simulink model "model_quarter_car_BG"  (Simulink 7.5)
settings: Solver=ode4  StartTime=0.0  StopTime=10  FixedStep=0.005  MaxStep=1e-6  RelTol=1e-3
settings Model: Creator=Slim  LastModifiedBy=Slim

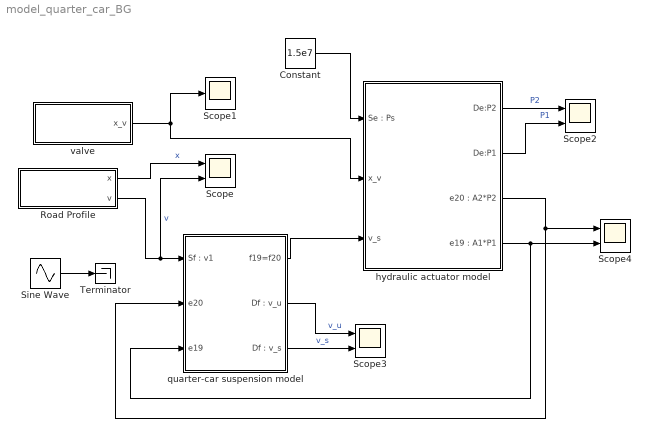
== system model_quarter_car_BG ==
  Constant : Constant  Value=1.5e7  OutDataType=fixdt(1, 16)  OutScaling=2^0
  Road Profile : Subsystem
  Scope{,2..4} (4 alike) : Scope  NumInputPorts=2
      Scope settings: YMin=-1~-5  YMax=1~5
      Scope2 settings: YMin=-1.25e+007~-5  YMax=1.25e+007~5  SaveName=ScopeData2
      Scope3 settings: YMin=-5~-5  YMax=5~5  SaveName=ScopeData3
      Scope4 settings: YMin=-1.25e+007~-5  YMax=1.25e+007~5  SaveName=ScopeData5
  Scope1 : Scope
      settings: YMin=6.25e-037  YMax=8.75e-037
  Sine Wave : Sin  Amplitude=0.08*pi  Bias=0  Frequency=2*pi  Phase=pi/2  Samples=10  SampleTime=0  Offset=0
  Terminator : Terminator
  hydraulic actuator model : Subsystem
  quarter-car suspension model : Subsystem
  valve : Subsystem
  wires:
  hydraulic actuator model/4("e19 : A1*P1") -> quarter-car suspension model/3(e19), Scope4/2
  hydraulic actuator model/3("e20 : A2*P2") -> quarter-car suspension model/2(e20), Scope4/1
  Road Profile/1(x) -> Scope/1  "x"
  valve/1(x_v) -> Scope1/1, hydraulic actuator model/2(x_v)
  Constant/1 -> hydraulic actuator model/1("Se : Ps")
  quarter-car suspension model/1(f19=f20) -> hydraulic actuator model/3(v_s)
  quarter-car suspension model/2("Df : v_u") -> Scope3/1  "v_u"
  quarter-car suspension model/3("Df : v_s") -> Scope3/2  "v_s"
  hydraulic actuator model/1(De:P2) -> Scope2/1  "P2"
  hydraulic actuator model/2(De:P1) -> Scope2/2  "P1"
  Sine Wave/1 -> Terminator/1
  Road Profile/2(v) -> quarter-car suspension model/1("Sf : v1"), Scope/2  "v"

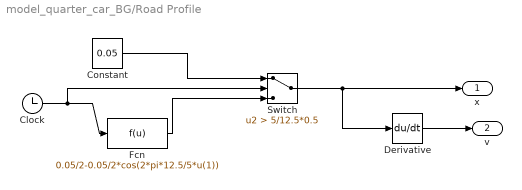
== system model_quarter_car_BG/Road Profile ==
  Clock : Clock
      settings: Decimation=10
  Constant : Constant  Value=0.05  OutDataType=fixdt(1, 16)  OutScaling=2^0
  Derivative : Derivative
  Fcn : Fcn  Expr=0.05/2-0.05/2*cos(2*pi*12.5/5*u(1))
  Switch : Switch  Criteria=u2 > Threshold  Threshold=5/12.5*0.5  OutDataType=fixdt(1, 16)  OutScaling=2^0
  x : Outport  OutDataType=fixdt(1, 16)  OutScaling=2^0
  v : Outport  Port=2  OutDataType=fixdt(1, 16)  OutScaling=2^0
  wires:
  Clock/1 -> Fcn/1, Switch/2
  Constant/1 -> Switch/1
  Fcn/1 -> Switch/3
  Switch/1 -> x/1, Derivative/1
  Derivative/1 -> v/1

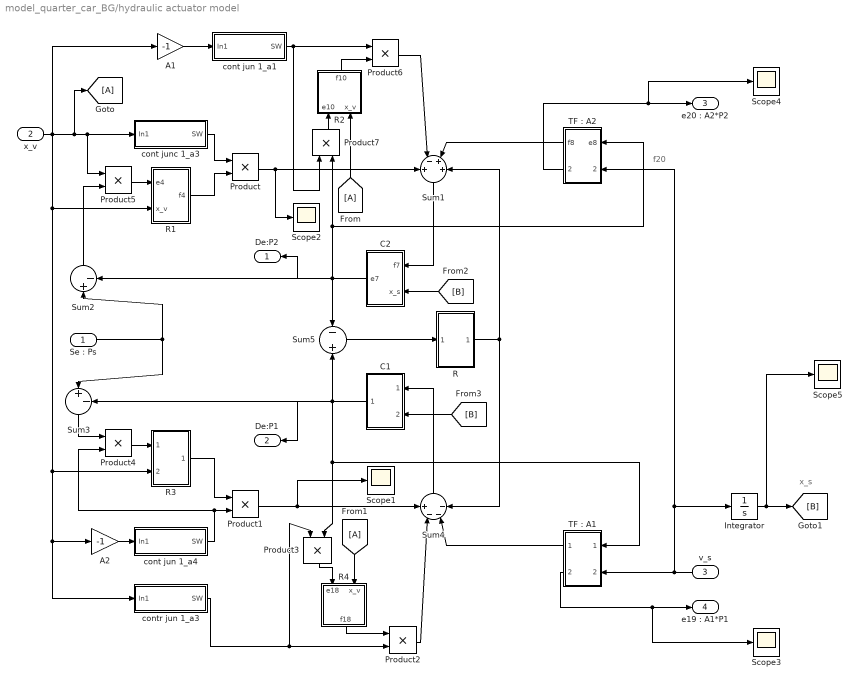
== system model_quarter_car_BG/hydraulic actuator model ==
  note: f20
  note: x_s
  "Se : Ps" : Inport  OutDataType=fixdt(1, 16)  OutScaling=2^0
  x_v : Inport  Port=2  OutDataType=fixdt(1, 16)  OutScaling=2^0
  v_s : Inport  Port=3  OutDataType=fixdt(1, 16)  OutScaling=2^0
  A1 : Gain  Gain=-1  ParameterDataType=fixdt(1, 16)  ParameterScaling=2^0  OutDataType=fixdt(1, 16)  OutScaling=2^0
  A2 : Gain  Gain=-1  ParameterDataType=fixdt(1, 16)  ParameterScaling=2^0  OutDataType=fixdt(1, 16)  OutScaling=2^0
  C1 : Subsystem
  C2 : Subsystem
  Integrator : Integrator
  Product{,1..7} (8 alike) : Product  OutDataType=fixdt(1, 16)  OutScaling=2^0  RndMeth=Zero
  R : Subsystem
  R1 : Subsystem
  R2 : Subsystem
  R3 : Subsystem
  R4 : Subsystem
  Scope{1..5} (5 alike) : Scope
      Scope1 settings: YMin=-1.25e+007  YMax=1.25e+007  SaveName=ScopeData6
      Scope2 settings: YMin=-1.25e+007  YMax=1.25e+007  SaveName=ScopeData4
      Scope3 settings: YMin=-1.25e+007  YMax=1.25e+007  SaveName=ScopeData8
      Scope4 settings: YMin=-1.25e+007  YMax=1.25e+007  SaveName=ScopeData9
      Scope5 settings: YMin=-1.25e+007  YMax=1.25e+007  SaveName=ScopeData10
  Sum1 : Sum  Inputs=+-++  OutDataType=fixdt(1, 16)  OutScaling=2^0
  Sum2 : Sum  Inputs=|+-  OutDataType=fixdt(1, 16)  OutScaling=2^0
  Sum3 : Sum  Inputs=|+-  OutDataType=fixdt(1, 16)  OutScaling=2^0
  Sum4 : Sum  Inputs=+---  OutDataType=fixdt(1, 16)  OutScaling=2^0
  Sum5 : Sum  Inputs=-+  OutDataType=fixdt(1, 16)  OutScaling=2^0
  "TF : A1" : Subsystem
  "TF : A2" : Subsystem
  cont jun 1_a1 : Subsystem
  cont jun 1_a4 : Subsystem
  cont junc 1_a3 : Subsystem
  contr jun 1_a3 : Subsystem
  De:P2 : Outport  OutDataType=fixdt(1, 16)  OutScaling=2^0
  De:P1 : Outport  Port=2  OutDataType=fixdt(1, 16)  OutScaling=2^0
  "e20 : A2*P2" : Outport  Port=3  OutDataType=fixdt(1, 16)  OutScaling=2^0
  "e19 : A1*P1" : Outport  Port=4  OutDataType=fixdt(1, 16)  OutScaling=2^0
  wires:
  "Se : Ps"/1 -> Sum2/1, Sum3/1
  cont junc 1_a3/1(SW) -> Product/1
  R1/1(f4) -> Product/2
  C2/1(e7) -> Sum2/2, Sum5/1, De:P2/1, "TF : A2"/1(e8), Product7/2
  Sum1/1 -> C2/1(f7)
  cont jun 1_a4/1(SW) -> Product1/2, Product4/2
  R3/1(f14) -> Product1/1
  Product/1 -> Sum1/1, Scope2/1
  C1/1(e16) -> Sum3/2, Sum5/2, De:P1/1, "TF : A1"/1(e17), Product3/2
  Sum4/1 -> C1/1(f16)
  Sum5/1 -> R/1(e11)
  Product1/1 -> Sum4/1, Scope1/1
  R/1(f11) -> Sum1/4, Sum4/4
  "TF : A2"/1(f8) -> Sum1/3
  "TF : A1"/1(f17) -> Sum4/3
  v_s/1 -> "TF : A1"/2(f19), "TF : A2"/2(f20), Integrator/1
  "TF : A1"/2(e19) -> "e19 : A1*P1"/1, Scope3/1
  "TF : A2"/2(e20) -> "e20 : A2*P2"/1, Scope4/1
  x_v/1 -> [A], cont junc 1_a3/1(In1), Product5/1, R3/2(x_v), A2/1, contr jun 1_a3/1(In1), R1/2(x_v), A1/1
  A2/1 -> cont jun 1_a4/1(In1)
  [A] -> R2/2(x_v)
  [A] -> R4/2(x_v)
  Integrator/1 -> [B], Scope5/1
  [B] -> C2/2(x_s)
  [B] -> C1/2(x_s)
  Sum2/1 -> Product5/2
  Sum3/1 -> Product4/1
  contr jun 1_a3/1(SW) -> Product2/2, Product3/1
  R4/1(f18) -> Product2/1
  Product2/1 -> Sum4/2
  Product3/1 -> R4/1(e18)
  Product4/1 -> R3/1(e14)
  Product5/1 -> R1/1(e4)
  A1/1 -> cont jun 1_a1/1(In1)
  cont jun 1_a1/1(SW) -> Product6/1, Product7/1
  R2/1(f10) -> Product6/2
  Product6/1 -> Sum1/2
  Product7/1 -> R2/1(e10)

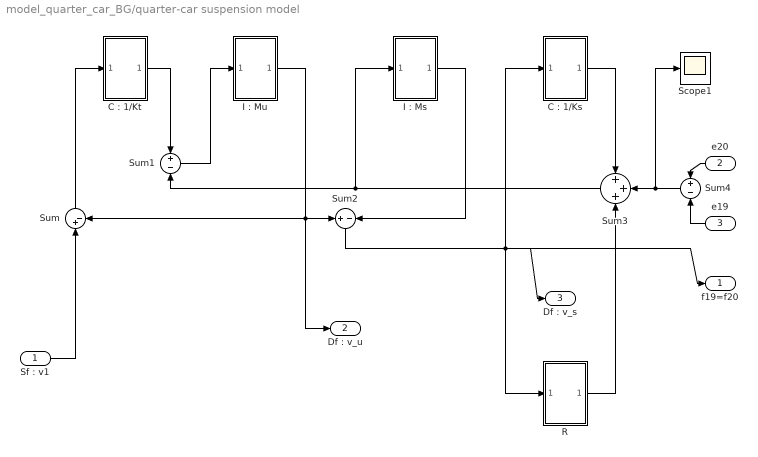
== system model_quarter_car_BG/quarter-car suspension model ==
  "Sf : v1" : Inport  OutDataType=fixdt(1, 16)  OutScaling=2^0
  e20 : Inport  Port=2  OutDataType=fixdt(1, 16)  OutScaling=2^0
  e19 : Inport  Port=3  OutDataType=fixdt(1, 16)  OutScaling=2^0
  "C : 1/Ks" : Subsystem
  "C : 1/Kt" : Subsystem
  "I : Ms" : Subsystem
  "I : Mu" : Subsystem
  R : Subsystem
  Scope1 : Scope
      settings: YMin=6.25e-037  YMax=8.75e-037  SaveName=ScopeData11
  Sum : Sum  Inputs=|+-  OutDataType=fixdt(1, 16)  OutScaling=2^0
  Sum1 : Sum  Inputs=+-  OutDataType=fixdt(1, 16)  OutScaling=2^0
  Sum2 : Sum  Inputs=+-  OutDataType=fixdt(1, 16)  OutScaling=2^0
  Sum3 : Sum  Inputs=+++  OutDataType=fixdt(1, 16)  OutScaling=2^0
  Sum4 : Sum  Inputs=+-  OutDataType=fixdt(1, 16)  OutScaling=2^0
  f19=f20 : Outport  OutDataType=fixdt(1, 16)  OutScaling=2^0
  "Df : v_u" : Outport  Port=2  OutDataType=fixdt(1, 16)  OutScaling=2^0
  "Df : v_s" : Outport  Port=3  OutDataType=fixdt(1, 16)  OutScaling=2^0
  wires:
  "Sf : v1"/1 -> Sum/1
  Sum/1 -> "C : 1/Kt"/1(f28)
  "C : 1/Kt"/1(e28) -> Sum1/1
  Sum1/1 -> "I : Mu"/1(e26)
  "I : Mu"/1(f26) -> Sum2/1, Sum/2, "Df : v_u"/1
  "I : Ms"/1(f24) -> Sum2/2
  Sum3/1 -> Sum1/2, "I : Ms"/1(e24)
  Sum2/1 -> "C : 1/Ks"/1(f21), R/1(f23), f19=f20/1, "Df : v_s"/1
  "C : 1/Ks"/1(e21) -> Sum3/1
  R/1(e23) -> Sum3/3
  e19/1 -> Sum4/2
  e20/1 -> Sum4/1
  Sum4/1 -> Sum3/2, Scope1/1

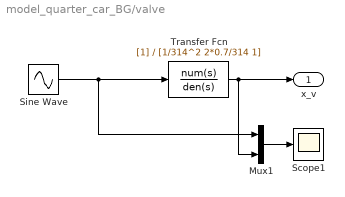
== system model_quarter_car_BG/valve ==
  Mux1 : Mux  Inputs=2
  Scope1 : Scope
      settings: YMin=6.25e-037  YMax=8.75e-037  SaveName=ScopeData7
  Sine Wave : Sin  Amplitude=2  Bias=0  Frequency=pi  Phase=0  Samples=10  SampleTime=0  Offset=0
  Transfer Fcn : TransferFcn  Denominator=[1/314^2 2*0.7/314 1]
  x_v : Outport  OutDataType=fixdt(1, 16)  OutScaling=2^0
  wires:
  Transfer Fcn/1 -> x_v/1, Mux1/2
  Sine Wave/1 -> Transfer Fcn/1, Mux1/1
  Mux1/1 -> Scope1/1

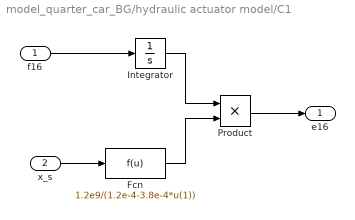
== system model_quarter_car_BG/hydraulic actuator model/C1 ==
  f16 : Inport  OutDataType=fixdt(1, 16)  OutScaling=2^0
  x_s : Inport  Port=2  OutDataType=fixdt(1, 16)  OutScaling=2^0
  Fcn : Fcn  Expr=1.2e9/(1.2e-4-3.8e-4*u(1))
  Integrator : Integrator
  Product : Product  OutDataType=fixdt(1, 16)  OutScaling=2^0  RndMeth=Zero
  e16 : Outport  OutDataType=fixdt(1, 16)  OutScaling=2^0
  wires:
  f16/1 -> Integrator/1
  Integrator/1 -> Product/1
  x_s/1 -> Fcn/1
  Fcn/1 -> Product/2
  Product/1 -> e16/1

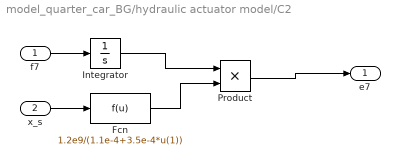
== system model_quarter_car_BG/hydraulic actuator model/C2 ==
  f7 : Inport  OutDataType=fixdt(1, 16)  OutScaling=2^0
  x_s : Inport  Port=2  OutDataType=fixdt(1, 16)  OutScaling=2^0
  Fcn : Fcn  Expr=1.2e9/(1.1e-4+3.5e-4*u(1))
  Integrator : Integrator
  Product : Product  OutDataType=fixdt(1, 16)  OutScaling=2^0  RndMeth=Zero
  e7 : Outport  OutDataType=fixdt(1, 16)  OutScaling=2^0
  wires:
  x_s/1 -> Fcn/1
  f7/1 -> Integrator/1
  Integrator/1 -> Product/1
  Fcn/1 -> Product/2
  Product/1 -> e7/1

== system model_quarter_car_BG/hydraulic actuator model/R ==
  e11 : Inport  OutDataType=fixdt(1, 16)  OutScaling=2^0
  1/Ctm : Gain  Gain=0.3e-12  ParameterDataType=fixdt(1, 16)  ParameterScaling=2^0  OutDataType=fixdt(1, 16)  OutScaling=2^0
  f11 : Outport  OutDataType=fixdt(1, 16)  OutScaling=2^0
  wires:
  e11/1 -> 1/Ctm/1
  1/Ctm/1 -> f11/1

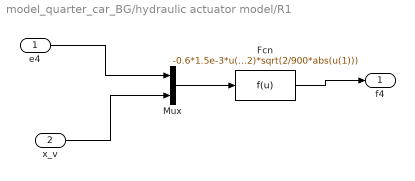
== system model_quarter_car_BG/hydraulic actuator model/R1 ==
  e4 : Inport  OutDataType=fixdt(1, 16)  OutScaling=2^0
  x_v : Inport  Port=2  OutDataType=fixdt(1, 16)  OutScaling=2^0
  Fcn : Fcn  Expr=-0.6*1.5e-3*u(2)*sqrt(2/900*abs(u(1)))
  Mux : Mux  Inputs=2
  f4 : Outport  OutDataType=fixdt(1, 16)  OutScaling=2^0
  wires:
  x_v/1 -> Mux/2
  e4/1 -> Mux/1
  Mux/1 -> Fcn/1
  Fcn/1 -> f4/1

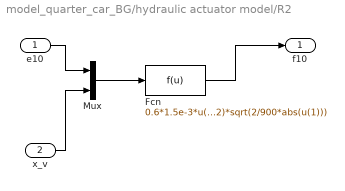
== system model_quarter_car_BG/hydraulic actuator model/R2 ==
  e10 : Inport  OutDataType=fixdt(1, 16)  OutScaling=2^0
  x_v : Inport  Port=2  OutDataType=fixdt(1, 16)  OutScaling=2^0
  Fcn : Fcn  Expr=0.6*1.5e-3*u(2)*sqrt(2/900*abs(u(1)))
  Mux : Mux  Inputs=2
  f10 : Outport  OutDataType=fixdt(1, 16)  OutScaling=2^0
  wires:
  e10/1 -> Mux/1
  x_v/1 -> Mux/2
  Mux/1 -> Fcn/1
  Fcn/1 -> f10/1

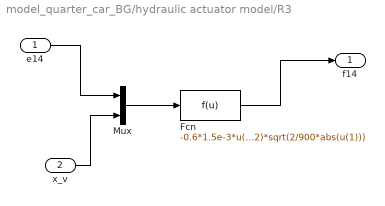
== system model_quarter_car_BG/hydraulic actuator model/R3 ==
  e14 : Inport  OutDataType=fixdt(1, 16)  OutScaling=2^0
  x_v : Inport  Port=2  OutDataType=fixdt(1, 16)  OutScaling=2^0
  Fcn : Fcn  Expr=-0.6*1.5e-3*u(2)*sqrt(2/900*abs(u(1)))
  Mux : Mux  Inputs=2
  f14 : Outport  OutDataType=fixdt(1, 16)  OutScaling=2^0
  wires:
  Mux/1 -> Fcn/1
  Fcn/1 -> f14/1
  e14/1 -> Mux/1
  x_v/1 -> Mux/2

== system model_quarter_car_BG/hydraulic actuator model/R4 ==
  e18 : Inport  OutDataType=fixdt(1, 16)  OutScaling=2^0
  x_v : Inport  Port=2  OutDataType=fixdt(1, 16)  OutScaling=2^0
  Fcn : Fcn  Expr=0.6*1.5e-3*u(2)*sqrt(2/900*abs(u(1)))
  Mux : Mux  Inputs=2
  f18 : Outport  OutDataType=fixdt(1, 16)  OutScaling=2^0
  wires:
  Fcn/1 -> f18/1
  Mux/1 -> Fcn/1
  e18/1 -> Mux/1
  x_v/1 -> Mux/2

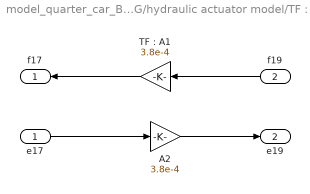
== system model_quarter_car_BG/hydraulic actuator model/TF : A1 ==
  e17 : Inport  OutDataType=fixdt(1, 16)  OutScaling=2^0
  f19 : Inport  Port=2  OutDataType=fixdt(1, 16)  OutScaling=2^0
  A2 : Gain  Gain=3.8e-4  ParameterDataType=fixdt(1, 16)  ParameterScaling=2^0  OutDataType=fixdt(1, 16)  OutScaling=2^0
  "TF : A1" : Gain  Gain=3.8e-4  ParameterDataType=fixdt(1, 16)  ParameterScaling=2^0  OutDataType=fixdt(1, 16)  OutScaling=2^0
  f17 : Outport  OutDataType=fixdt(1, 16)  OutScaling=2^0
  e19 : Outport  Port=2  OutDataType=fixdt(1, 16)  OutScaling=2^0
  wires:
  A2/1 -> e19/1
  e17/1 -> A2/1
  "TF : A1"/1 -> f17/1
  f19/1 -> "TF : A1"/1

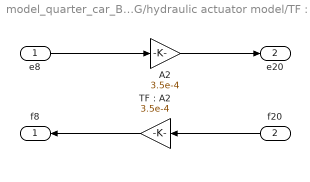
== system model_quarter_car_BG/hydraulic actuator model/TF : A2 ==
  e8 : Inport  OutDataType=fixdt(1, 16)  OutScaling=2^0
  f20 : Inport  Port=2  OutDataType=fixdt(1, 16)  OutScaling=2^0
  A2 : Gain  Gain=3.5e-4  ParameterDataType=fixdt(1, 16)  ParameterScaling=2^0  OutDataType=fixdt(1, 16)  OutScaling=2^0
  "TF : A2" : Gain  Gain=3.5e-4  ParameterDataType=fixdt(1, 16)  ParameterScaling=2^0  OutDataType=fixdt(1, 16)  OutScaling=2^0
  f8 : Outport  OutDataType=fixdt(1, 16)  OutScaling=2^0
  e20 : Outport  Port=2  OutDataType=fixdt(1, 16)  OutScaling=2^0
  wires:
  f20/1 -> "TF : A2"/1
  "TF : A2"/1 -> f8/1
  e8/1 -> A2/1
  A2/1 -> e20/1

== system model_quarter_car_BG/hydraulic actuator model/cont jun 1_a1 ==
  In1 : Inport  OutDataType=fixdt(1, 16)  OutScaling=2^0
  Constant : Constant  OutDataType=sfix(16)  OutScaling=2^0
  Constant1 : Constant  Value=0  OutDataType=sfix(16)  OutScaling=2^0
  Switch : Switch  Criteria=u2 > Threshold  OutDataType=sfix(16)  OutScaling=2^0
  SW : Outport  OutDataType=fixdt(1, 16)  OutScaling=2^0
  wires:
  Switch/1 -> SW/1
  Constant/1 -> Switch/1
  Constant1/1 -> Switch/3
  In1/1 -> Switch/2

== system model_quarter_car_BG/hydraulic actuator model/cont jun 1_a4 ==
  In1 : Inport  OutDataType=fixdt(1, 16)  OutScaling=2^0
  Constant : Constant  OutDataType=sfix(16)  OutScaling=2^0
  Constant1 : Constant  Value=0  OutDataType=sfix(16)  OutScaling=2^0
  Switch : Switch  Criteria=u2 > Threshold  OutDataType=sfix(16)  OutScaling=2^0
  SW : Outport  OutDataType=fixdt(1, 16)  OutScaling=2^0
  wires:
  In1/1 -> Switch/2
  Constant1/1 -> Switch/3
  Constant/1 -> Switch/1
  Switch/1 -> SW/1

== system model_quarter_car_BG/hydraulic actuator model/cont junc 1_a3 ==
  In1 : Inport  OutDataType=fixdt(1, 16)  OutScaling=2^0
  Constant : Constant  OutDataType=sfix(16)  OutScaling=2^0
  Constant1 : Constant  Value=0  OutDataType=sfix(16)  OutScaling=2^0
  Switch : Switch  OutDataType=sfix(16)  OutScaling=2^0
  SW : Outport  OutDataType=fixdt(1, 16)  OutScaling=2^0
  wires:
  Switch/1 -> SW/1
  Constant/1 -> Switch/1
  Constant1/1 -> Switch/3
  In1/1 -> Switch/2

== system model_quarter_car_BG/hydraulic actuator model/contr jun 1_a3 ==
  In1 : Inport  OutDataType=fixdt(1, 16)  OutScaling=2^0
  Constant : Constant  OutDataType=sfix(16)  OutScaling=2^0
  Constant1 : Constant  Value=0  OutDataType=sfix(16)  OutScaling=2^0
  Switch : Switch  OutDataType=sfix(16)  OutScaling=2^0
  SW : Outport  OutDataType=fixdt(1, 16)  OutScaling=2^0
  wires:
  In1/1 -> Switch/2
  Constant1/1 -> Switch/3
  Constant/1 -> Switch/1
  Switch/1 -> SW/1

== system model_quarter_car_BG/quarter-car suspension model/C : 1/Ks ==
  f21 : Inport  OutDataType=fixdt(1, 16)  OutScaling=2^0
  1/C1 : Gain  Gain=16800  ParameterDataType=fixdt(1, 16)  ParameterScaling=2^0  OutDataType=fixdt(1, 16)  OutScaling=2^0
  Integrator : Integrator
  e21 : Outport  OutDataType=fixdt(1, 16)  OutScaling=2^0
  wires:
  1/C1/1 -> e21/1
  Integrator/1 -> 1/C1/1
  f21/1 -> Integrator/1

== system model_quarter_car_BG/quarter-car suspension model/C : 1/Kt ==
  f28 : Inport  OutDataType=fixdt(1, 16)  OutScaling=2^0
  1/C1 : Gain  Gain=190000  ParameterDataType=fixdt(1, 16)  ParameterScaling=2^0  OutDataType=fixdt(1, 16)  OutScaling=2^0
  Integrator : Integrator
  e28 : Outport  OutDataType=fixdt(1, 16)  OutScaling=2^0
  wires:
  f28/1 -> Integrator/1
  Integrator/1 -> 1/C1/1
  1/C1/1 -> e28/1

== system model_quarter_car_BG/quarter-car suspension model/I : Ms ==
  e24 : Inport  OutDataType=fixdt(1, 16)  OutScaling=2^0
  1/I : Gain  Gain=1/290  ParameterDataType=fixdt(1, 16)  ParameterScaling=2^0  OutDataType=fixdt(1, 16)  OutScaling=2^0
  Integrator : Integrator
  f24 : Outport  OutDataType=fixdt(1, 16)  OutScaling=2^0
  wires:
  1/I/1 -> f24/1
  Integrator/1 -> 1/I/1
  e24/1 -> Integrator/1

== system model_quarter_car_BG/quarter-car suspension model/I : Mu ==
  e26 : Inport  OutDataType=fixdt(1, 16)  OutScaling=2^0
  1/I : Gain  Gain=1/59  ParameterDataType=fixdt(1, 16)  ParameterScaling=2^0  OutDataType=fixdt(1, 16)  OutScaling=2^0
  Integrator : Integrator
  f26 : Outport  OutDataType=fixdt(1, 16)  OutScaling=2^0
  wires:
  e26/1 -> Integrator/1
  Integrator/1 -> 1/I/1
  1/I/1 -> f26/1

== system model_quarter_car_BG/quarter-car suspension model/R ==
  f23 : Inport  OutDataType=fixdt(1, 16)  OutScaling=2^0
  R : Gain  Gain=1000  ParameterDataType=fixdt(1, 16)  ParameterScaling=2^0  OutDataType=fixdt(1, 16)  OutScaling=2^0
  e23 : Outport  OutDataType=fixdt(1, 16)  OutScaling=2^0
  wires:
  R/1 -> e23/1
  f23/1 -> R/1
